simulink model "OBC_dataprocessing"  (R2021b)
settings: Solver=VariableStepAuto  StartTime=0.0  StopTime=10.0  RelTol=1e-3
values from neighbouring files (symbols this model uses):
  V_test = [Vxp,Vxn,Vyp,Vyn]    [DAL_Declarations.m]
undefined symbols (not defined in the file or in its folder): magnitude
settings Model: Creator=Andrea  LastModifiedBy=Andrea

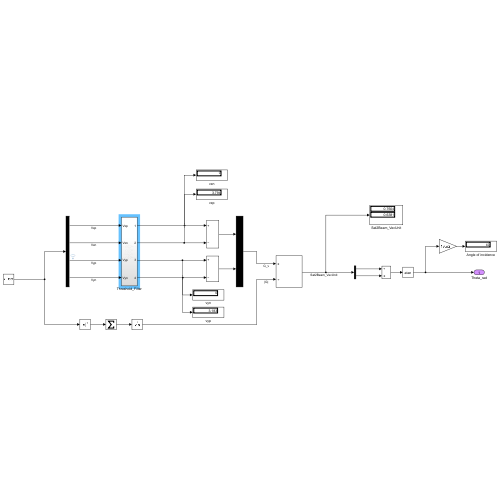
[thumbnail: Simulink's stored preview of the top-level diagram]
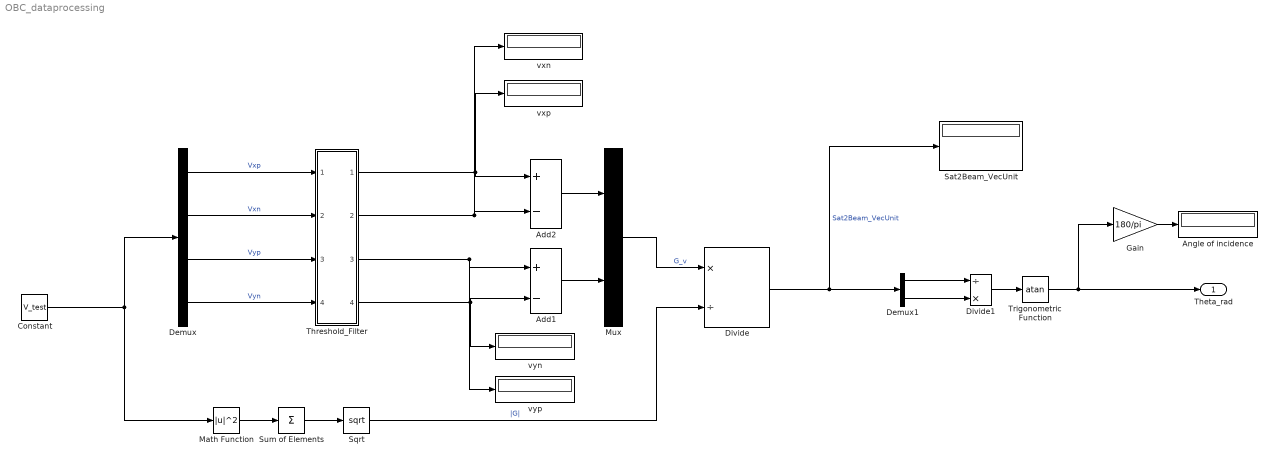
== system OBC_dataprocessing ==
  Add1 : Sum  Inputs=+|-
  Add2 : Sum  Inputs=+|-
  Angle of incidence : Display
  Constant : Constant  Value=V_test
  Demux : Demux
  Demux1 : Demux  Outputs=2
  Divide : Product  Inputs=*/
  Divide1 : Product  Inputs=/*
  Gain : Gain  Gain=180/pi
  Math Function : Math  Operator=magnitude^2  OutputSignalType=real  SaturateOnIntegerOverflow=on
  Mux : Mux  Inputs=2
  Sat2Beam_VecUnit : Display
  Sqrt : Sqrt  SaturateOnIntegerOverflow=on
  Sum of Elements : Sum  Inputs=+
  Threshold_Filter : Subsystem
  Trigonometric Function : Trigonometry  Operator=atan
  vxn : Display
  vxp : Display
  vyn : Display
  vyp : Display
  Theta_rad : Outport
  wires:
  Sqrt/1 -> Divide/2  "|G|"
  Math Function/1 -> Sum of Elements/1
  Add2/1 -> Mux/1
  Demux/4 -> Threshold_Filter/4(Vyn)  "Vyn"
  Trigonometric Function/1 -> Gain/1, Theta_rad/1
  Demux1/1 -> Divide1/1
  Constant/1 -> Math Function/1, Demux/1
  Mux/1 -> Divide/1  "G_v"
  Add1/1 -> Mux/2
  Divide1/1 -> Trigonometric Function/1
  Divide/1 -> Demux1/1, Sat2Beam_VecUnit/1  "Sat2Beam_VecUnit"
  Sum of Elements/1 -> Sqrt/1
  Demux/3 -> Threshold_Filter/3(Vyp)  "Vyp"
  Demux1/2 -> Divide1/2
  Gain/1 -> Angle of incidence/1
  Demux/2 -> Threshold_Filter/2(Vxn)  "Vxn"
  Demux/1 -> Threshold_Filter/1(Vxp)  "Vxp"
  Threshold_Filter/4(Out4) -> vyn/1, Add1/2
  Threshold_Filter/1(Out1) -> vxp/1, Add2/1
  Threshold_Filter/2(Out2) -> Add2/2, vxn/1
  Threshold_Filter/3(Out3) -> vyp/1, Add1/1

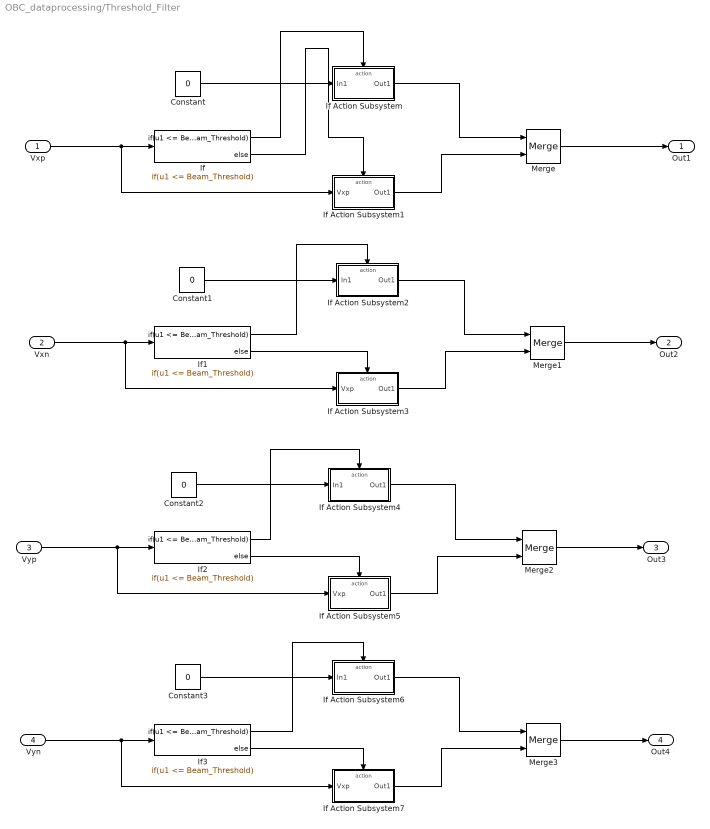
== system OBC_dataprocessing/Threshold_Filter ==
  Vxp : Inport
  Vxn : Inport  Port=2
  Vyp : Inport  Port=3
  Vyn : Inport  Port=4
  Constant{,1..3} (4 alike) : Constant  Value=0
  If{,1..3} (4 alike) : If  IfExpression=u1 <= Beam_Threshold
  If Action Subsystem : Subsystem  TreatAsAtomicUnit=on
  If Action Subsystem1 : Subsystem  TreatAsAtomicUnit=on
  If Action Subsystem2 : Subsystem  TreatAsAtomicUnit=on
  If Action Subsystem3 : Subsystem  TreatAsAtomicUnit=on
  If Action Subsystem4 : Subsystem  TreatAsAtomicUnit=on
  If Action Subsystem5 : Subsystem  TreatAsAtomicUnit=on
  If Action Subsystem6 : Subsystem  TreatAsAtomicUnit=on
  If Action Subsystem7 : Subsystem  TreatAsAtomicUnit=on
  Merge{,1..3} (4 alike) : Merge
  Out1 : Outport
  Out2 : Outport  Port=2
  Out3 : Outport  Port=3
  Out4 : Outport  Port=4
  wires:
  Vxp/1 -> If Action Subsystem1/1(Vxp), If/1
  If/1 -> If Action Subsystem/Action
  If Action Subsystem/1(Out1) -> Merge/1
  If/2 -> If Action Subsystem1/Action
  If Action Subsystem1/1(Out1) -> Merge/2
  Merge/1 -> Out1/1
  Constant/1 -> If Action Subsystem/1(In1)
  If Action Subsystem3/1(Out1) -> Merge1/2
  Constant1/1 -> If Action Subsystem2/1(In1)
  If1/1 -> If Action Subsystem2/Action
  Vxn/1 -> If1/1, If Action Subsystem3/1(Vxp)
  If Action Subsystem2/1(Out1) -> Merge1/1
  If1/2 -> If Action Subsystem3/Action
  Merge1/1 -> Out2/1
  Vyp/1 -> If2/1, If Action Subsystem5/1(Vxp)
  If2/2 -> If Action Subsystem5/Action
  If2/1 -> If Action Subsystem4/Action
  If Action Subsystem4/1(Out1) -> Merge2/1
  If Action Subsystem5/1(Out1) -> Merge2/2
  Constant2/1 -> If Action Subsystem4/1(In1)
  Merge2/1 -> Out3/1
  Vyn/1 -> If3/1, If Action Subsystem7/1(Vxp)
  Merge3/1 -> Out4/1
  If Action Subsystem7/1(Out1) -> Merge3/2
  If3/2 -> If Action Subsystem7/Action
  If Action Subsystem6/1(Out1) -> Merge3/1
  Constant3/1 -> If Action Subsystem6/1(In1)
  If3/1 -> If Action Subsystem6/Action

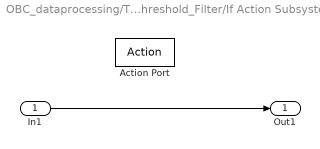
== system OBC_dataprocessing/Threshold_Filter/If Action Subsystem ==
  In1 : Inport
  Action Port : ActionPort  ActionPortLabel=if(u1 < Beam_Threshold)
  Out1 : Outport
  wires:
  In1/1 -> Out1/1

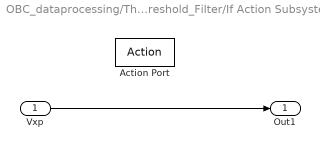
== system OBC_dataprocessing/Threshold_Filter/If Action Subsystem1 ==
  Vxp : Inport
  Action Port : ActionPort  ActionPortLabel=else
  Out1 : Outport
  wires:
  Vxp/1 -> Out1/1

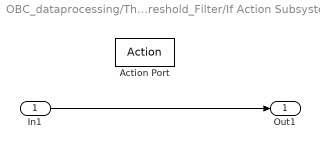
== system OBC_dataprocessing/Threshold_Filter/If Action Subsystem2 ==
  In1 : Inport
  Action Port : ActionPort  ActionPortLabel=if(u1 < Beam_Threshold)
  Out1 : Outport
  wires:
  In1/1 -> Out1/1

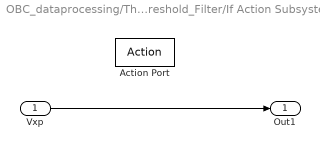
== system OBC_dataprocessing/Threshold_Filter/If Action Subsystem3 ==
  Vxp : Inport
  Action Port : ActionPort  ActionPortLabel=else
  Out1 : Outport
  wires:
  Vxp/1 -> Out1/1

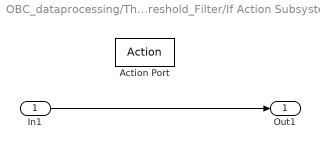
== system OBC_dataprocessing/Threshold_Filter/If Action Subsystem4 ==
  In1 : Inport
  Action Port : ActionPort  ActionPortLabel=if(u1 < Beam_Threshold)
  Out1 : Outport
  wires:
  In1/1 -> Out1/1

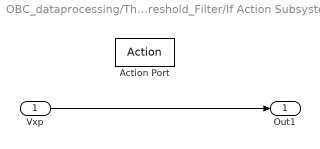
== system OBC_dataprocessing/Threshold_Filter/If Action Subsystem5 ==
  Vxp : Inport
  Action Port : ActionPort  ActionPortLabel=else
  Out1 : Outport
  wires:
  Vxp/1 -> Out1/1

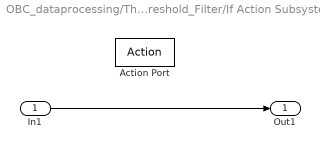
== system OBC_dataprocessing/Threshold_Filter/If Action Subsystem6 ==
  In1 : Inport
  Action Port : ActionPort  ActionPortLabel=if(u1 < Beam_Threshold)
  Out1 : Outport
  wires:
  In1/1 -> Out1/1

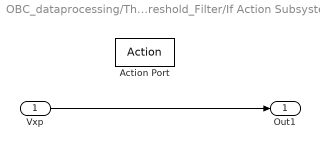
== system OBC_dataprocessing/Threshold_Filter/If Action Subsystem7 ==
  Vxp : Inport
  Action Port : ActionPort  ActionPortLabel=else
  Out1 : Outport
  wires:
  Vxp/1 -> Out1/1
